simulink model "SPGF_FSK_0000_R2020b"  (R2020b)
settings: Solver=ode4  StartTime=0.0  StopTime=1.4  FixedStep=50e-6/50  RelTol=1e-3  EnableMultiTasking=on
undefined symbols (not defined in the file): D11, Delta
libraries: powerlib x2546, powerlib_meascontrol x183, simulink x24
(part 11 of 34)

== system SPGF_FSK_0000_R2020b/V53/VT ==
  Ground3 : powerlib/Elements/Ground  LConnTagsString=a
  Ground4 : powerlib/Elements/Ground  LConnTagsString=a
  Ground5 : powerlib/Elements/Ground  LConnTagsString=a
  Mux2 : Mux  Inputs=3
  Mux3 : Mux  Inputs=3
  R Load A1 : powerlib/Elements/Series RLC Load  LConnTagsString=a  RConnTagsString=__new0  NominalVoltage=57.735  NominalFrequency=50  ActivePower=150  InductivePower=0  CapacitivePower=0  Setx0=off  InitialVoltage=0  SetiL0=off  InitialCurrent=0  Measurements=None  LoadType=constant Z
  R Load B1 : powerlib/Elements/Series RLC Load  LConnTagsString=a  RConnTagsString=__new0  NominalVoltage=57.735  NominalFrequency=50  ActivePower=150  InductivePower=0  CapacitivePower=0  Setx0=off  InitialVoltage=0  SetiL0=off  InitialCurrent=0  Measurements=None  LoadType=constant Z
  R Load C1 : powerlib/Elements/Series RLC Load  LConnTagsString=a  RConnTagsString=__new0  NominalVoltage=57.735  NominalFrequency=50  ActivePower=150  InductivePower=0  CapacitivePower=0  Setx0=off  InitialVoltage=0  SetiL0=off  InitialCurrent=0  Measurements=None  LoadType=constant Z
  U A:3 : powerlib/Measurements/Voltage Measurement  PhasorSimulation=off  OutputType=Complex  PSBequivalent=0
  U A:4 : powerlib/Measurements/Voltage Measurement  PhasorSimulation=off  OutputType=Complex  PSBequivalent=0
  U B:3 : powerlib/Measurements/Voltage Measurement  PhasorSimulation=off  OutputType=Complex  PSBequivalent=0
  U B:4 : powerlib/Measurements/Voltage Measurement  PhasorSimulation=off  OutputType=Complex  PSBequivalent=0
  U C:3 : powerlib/Measurements/Voltage Measurement  PhasorSimulation=off  OutputType=Complex  PSBequivalent=0
  U C:4 : powerlib/Measurements/Voltage Measurement  PhasorSimulation=off  OutputType=Complex  PSBequivalent=0
  U0:1 : powerlib/Measurements/Voltage Measurement  PhasorSimulation=off  OutputType=Complex  PSBequivalent=0
  VT A1 : powerlib/Elements/Saturable Transformer  ThreeWindings=on  Hysteresis=off  DataFile='hysteresis.mat'  Measurements=None  UNITS=pu  NominalPower=[600, 50]  Winding1=[5773.503, 0.00562500, 0.02315000]  Winding2=[57.735, 0.00562500, 0.02315000]  Winding3=[33.333, 0.00010000, 0.00010000]  Saturation=[ 0,0 ; 0.0024,1.2 ; 1.0,1.52 ]  CoreLoss=[500]  BreakLoop=on  DiscreteSolver=Trapezoidal iterative  DataType=off  InitialFlux=-24.6148264896066  TransfoNumber=1
  VT B1 : powerlib/Elements/Saturable Transformer  ThreeWindings=on  Hysteresis=off  DataFile='hysteresis.mat'  Measurements=None  UNITS=pu  NominalPower=[600, 50]  Winding1=[5773.503, 0.00562500, 0.02315000]  Winding2=[57.735, 0.00562500, 0.02315000]  Winding3=[33.333, 0.00010000, 0.00010000]  Saturation=[ 0,0 ; 0.0024,1.2 ; 1.0,1.52 ]  CoreLoss=[500]  BreakLoop=on  DiscreteSolver=Trapezoidal iterative  DataType=off  InitialFlux=0.429801202991945  TransfoNumber=1
  VT C1 : powerlib/Elements/Saturable Transformer  ThreeWindings=on  Hysteresis=off  DataFile='hysteresis.mat'  Measurements=None  UNITS=pu  NominalPower=[600, 50]  Winding1=[5773.503, 0.00562500, 0.02315000]  Winding2=[57.735, 0.00562500, 0.02315000]  Winding3=[33.333, 0.00010000, 0.00010000]  Saturation=[ 0,0 ; 0.0024,1.2 ; 1.0,1.52 ]  CoreLoss=[500]  BreakLoop=on  DiscreteSolver=Trapezoidal iterative  DataType=off  InitialFlux=24.1850252874139  TransfoNumber=1
  A : PMIOPort  Side=Left
  B : PMIOPort  Port=2  Side=Left
  C : PMIOPort  Port=3  Side=Left
  Uabc1 : Outport
  Uabc2 : Outport  Port=2
  3U0 : Outport  Port=3
  wires:
  Mux3/1 -> Uabc2/1
  U0:1/1 -> 3U0/1
  Mux2/1 -> Uabc1/1
  U C:4/1 -> Mux3/3
  U B:4/1 -> Mux3/2
  U A:4/1 -> Mux3/1
  U C:3/1 -> Mux2/3
  U B:3/1 -> Mux2/2
  U A:3/1 -> Mux2/1
  connections:
  VT C1/RConn4 -- U0:1/LConn2 -- Ground4/LConn1
  U A:4/LConn2 -- U B:4/LConn2 -- U C:4/LConn2 -- R Load A1/RConn1 -- R Load B1/RConn1 -- R Load C1/RConn1 -- VT C1/RConn2 -- VT B1/RConn2 -- VT A1/RConn2
  VT B1/RConn1 -- R Load B1/LConn1 -- U B:4/LConn1
  VT C1/RConn1 -- R Load C1/LConn1 -- U C:4/LConn1
  VT B1/LConn1 -- U B:3/LConn1 -- B/RConn1
  VT C1/LConn1 -- U C:3/LConn1 -- C/RConn1
  VT A1/RConn1 -- R Load A1/LConn1 -- U A:4/LConn1
  U A:3/LConn1 -- VT A1/LConn1 -- A/RConn1
  Ground3/LConn1 -- U C:3/LConn2 -- VT B1/LConn2 -- U B:3/LConn2 -- VT A1/LConn2 -- U A:3/LConn2 -- VT C1/LConn2
  VT B1/RConn4 -- VT C1/RConn3
  VT A1/RConn3 -- U0:1/LConn1
  VT A1/RConn4 -- VT B1/RConn3
